simulink model "sf_newtons_cradle_vr"  (R2017b)
settings: Solver=ode45  StartTime=0.0  StopTime=inf  RelTol=1e-3
libraries: vrlib x3
settings Model: Creator=The MathWorks, Inc.  LastModifiedBy=The MathWorks, Inc.
settings DataIOCC: LimitDataPoints=on  SaveFormat=Array
settings OptimizationCC: BlockReduction=off  ExpressionDepthLimit=2147483647  InitFltsAndDblsToZero=on  LifeSpan=inf
settings DebuggingCC: UnderspecifiedInitializationDetection=Classic  MergeDetectMultiDrivingBlocksExec=none  SignalResolutionControl=TryResolveAllWithWarning  FcnCallInpInsideContextMsg=warning  StateNameClashWarn=warning  StrictBusMsg=Warning  SFUnexpectedBacktrackingDiag=warning  SFNoUnconditionalDefaultTransitionDiag=warning  SFExecutionAtInitializationDiag=none
settings HardwareCC: ProdBitPerPointer=32  ProdBitPerSizeT=32  ProdBitPerPtrDiffT=32  ProdLargestAtomicFloat=None  ProdIntDivRoundTo=Undefined  ProdEndianess=Unspecified  ProdWordSize=32  ProdHWDeviceType=32-bit Generic  TargetUnknown=on
settings ModelReferenceCC: PropagateSignalLabelsOutOfModel=off
settings SFSimCC: SFSimEcho=off  SimParseCustomCode=off
settings CodeAppCC: StateflowObjectComments=on
settings GRTTargetCC: TargetFcnLib=ansi_tfl_tmw_new.mat  TargetLangStandard=C89/C90 (ANSI)  GeneratePreprocessorConditionals=Disable all  CombineOutputUpdateFcns=off  GRTInterface=on
settings ConfigComp: CovMetricSettings=dw  CovHtmlReporting=on  CovSaveCumulativeToWorkspaceVar=on  CovSaveSingleToWorkspaceVar=on  CovExternalEMLEnable=off  CovSFcnEnable=off

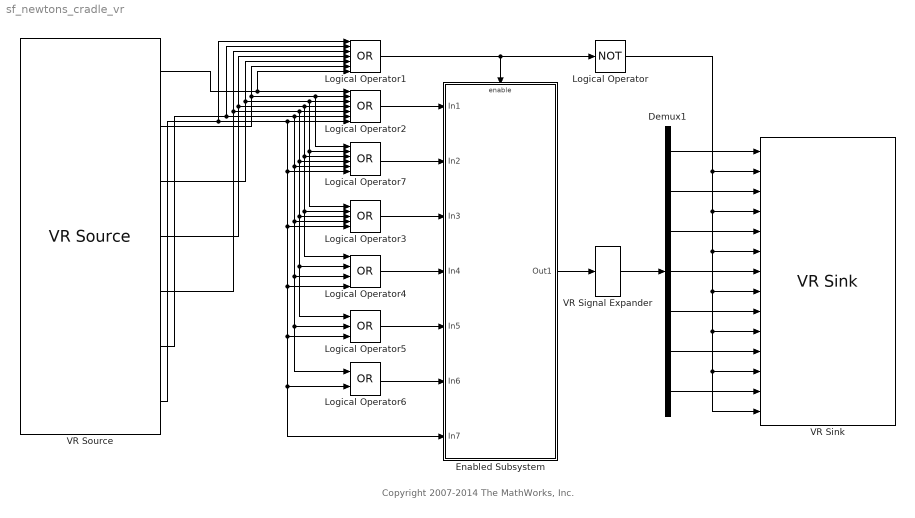
== system sf_newtons_cradle_vr ==
  note: Copyright 2007-2014 The MathWorks, Inc.
  Demux1 : Demux  Outputs=7
  Enabled Subsystem : Subsystem  TreatAsAtomicUnit=on
  Logical Operator : Logic  Operator=NOT  AllPortsSameDT=off  OutDataTypeStr=boolean
  Logical Operator1 : Logic  Operator=OR  Inputs=7  AllPortsSameDT=off  OutDataTypeStr=boolean
  Logical Operator2 : Logic  Operator=OR  Inputs=7  AllPortsSameDT=off  OutDataTypeStr=boolean
  Logical Operator3 : Logic  Operator=OR  Inputs=5  AllPortsSameDT=off  OutDataTypeStr=boolean
  Logical Operator4 : Logic  Operator=OR  Inputs=4  AllPortsSameDT=off  OutDataTypeStr=boolean
  Logical Operator5 : Logic  Operator=OR  Inputs=3  AllPortsSameDT=off  OutDataTypeStr=boolean
  Logical Operator6 : Logic  Operator=OR  AllPortsSameDT=off  OutDataTypeStr=boolean
  Logical Operator7 : Logic  Operator=OR  Inputs=6  AllPortsSameDT=off  OutDataTypeStr=boolean
  VR Signal Expander : vrlib/VR Signal Expander  outwidth=28  outidx=[4 8 12 16 20 24 28]
      settings: SourceProductName=Simulink 3D Animation  SourceProductBaseCode=VR
  VR Sink : vrlib/VR Sink  InstantiateOnLoad=on  SampleTime=0.01  ViewEnable=on  RemoteChange=off  RemoteView=off  FieldsWritten=Assembly1.ProtoRotation.4.1.1.double#Assembly1.ProtoEnabled.1.1.1.logical#Assembly2.ProtoRotation.4.1.1.double#Assembly2.ProtoEnabled.1.1.1.logical#Assembly3.ProtoRotation.4.1.1.double#Assembly3.ProtoEnabled.1.1.1.logical#Assembly4.ProtoRotation.4.1.1.double#Assembly4.ProtoEnabled.1.1.1.logical#Assembly5.ProtoRotation.4.1.1.double#Assembly5.ProtoEnabled.1.1.1.logical#Assembly6.ProtoRotation.4.1.1.double#Assembly6.ProtoEnabled.1.1.1.logical#Assembly7.ProtoRotation.4.1.1.double#Assembly7.ProtoEnabled.1.1.1.logical  WorldFileName=cradle.wrl  AutoView=off  VideoDimensions=[]  AllowVariableSize=off
      settings: SourceProductBaseCode=VR
  VR Source : vrlib/VR Source  InstantiateOnLoad=on  SampleTime=0.1  ViewEnable=on  RemoteChange=off  RemoteView=off  FieldsRead=Assembly1.ProtoIsActive.1.1.1.logical#Assembly2.ProtoIsActive.1.1.1.logical#Assembly3.ProtoIsActive.1.1.1.logical#Assembly4.ProtoIsActive.1.1.1.logical#Assembly5.ProtoIsActive.1.1.1.logical#Assembly6.ProtoIsActive.1.1.1.logical#Assembly7.ProtoIsActive.1.1.1.logical  WorldFileName=cradle.wrl  AutoView=off  VideoDimensions=[]  AllowVariableSize=off
      settings: SourceProductName=Simulink 3D Animation  SourceProductBaseCode=VR
  wires:
  Demux1/1 -> VR Sink/1
  Demux1/2 -> VR Sink/3
  Demux1/3 -> VR Sink/5
  Demux1/4 -> VR Sink/7
  Demux1/5 -> VR Sink/9
  Demux1/6 -> VR Sink/11
  Demux1/7 -> VR Sink/13
  Logical Operator/1 -> VR Sink/2, VR Sink/8, VR Sink/14, VR Sink/12, VR Sink/10, VR Sink/6, VR Sink/4
  VR Signal Expander/1 -> Demux1/1
  Logical Operator1/1 -> Logical Operator/1, Enabled Subsystem/Enable
  VR Source/1 -> Logical Operator1/7, Logical Operator2/1
  VR Source/2 -> Logical Operator1/6, Logical Operator2/2, Logical Operator7/1
  VR Source/3 -> Logical Operator1/5, Logical Operator3/1, Logical Operator7/2, Logical Operator2/3
  VR Source/4 -> Logical Operator1/4, Logical Operator4/1, Logical Operator3/2, Logical Operator7/3, Logical Operator2/4
  VR Source/5 -> Logical Operator1/3, Logical Operator5/1, Logical Operator4/2, Logical Operator3/3, Logical Operator7/4, Logical Operator2/5
  Logical Operator2/1 -> Enabled Subsystem/1(In1)
  Logical Operator7/1 -> Enabled Subsystem/2(In2)
  Logical Operator3/1 -> Enabled Subsystem/3(In3)
  Logical Operator4/1 -> Enabled Subsystem/4(In4)
  Logical Operator5/1 -> Enabled Subsystem/5(In5)
  Logical Operator6/1 -> Enabled Subsystem/6(In6)
  VR Source/6 -> Logical Operator1/2, Logical Operator6/1, Logical Operator5/2, Logical Operator4/3, Logical Operator3/4, Logical Operator7/5, Logical Operator2/6
  VR Source/7 -> Logical Operator1/1, Enabled Subsystem/7(In7), Logical Operator6/2, Logical Operator5/3, Logical Operator4/4, Logical Operator3/5, Logical Operator7/6, Logical Operator2/7
  Enabled Subsystem/1(Out1) -> VR Signal Expander/1

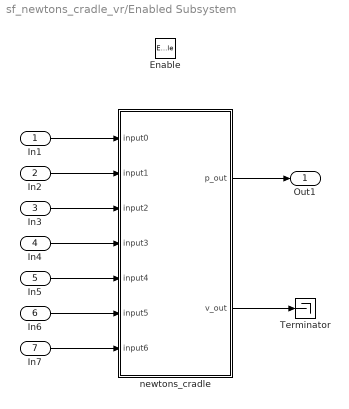
== system sf_newtons_cradle_vr/Enabled Subsystem ==
  In1 : Inport
  In2 : Inport  Port=2
  In3 : Inport  Port=3
  In4 : Inport  Port=4
  In5 : Inport  Port=5
  In6 : Inport  Port=6
  In7 : Inport  Port=7
  Enable : EnablePort
  Terminator : Terminator
  newtons_cradle : Stateflow chart  TreatAsAtomicUnit=on
  Out1 : Outport
  wires:
  newtons_cradle/2(v_out) -> Terminator/1
  newtons_cradle/1(p_out) -> Out1/1
  In3/1 -> newtons_cradle/3(input2)
  In4/1 -> newtons_cradle/4(input3)
  In2/1 -> newtons_cradle/2(input1)
  In1/1 -> newtons_cradle/1(input0)
  In5/1 -> newtons_cradle/5(input4)
  In6/1 -> newtons_cradle/6(input5)
  In7/1 -> newtons_cradle/7(input6)

== stateflow chart sf_newtons_cradle_vr/Enabled Subsystem/newtons_cradle ==
  settings: updateMethod=CONTINUOUS  initializeOutput=1
  state FreeDynamics
    du:
    p_out = p;
    v_out = v;
    p_dot = v;
    v_dot = -g/l*sin(p);
  state resetPositionsAndVelocities [function]
    (default) -> (junction 22) : {i=0;}
    (junction 22) -> (junction 24) [order 1] : [i < k-1]
    (junction 17) -> (junction 22) : {i++;}
    (junction 24) -> (junction 17) [order 2]
    (junction 24) -> (junction 17) [order 1] : [p[i] < p[i+1]]
        | {
        | // swap positions
        | tmp = p[i];
        | p[i] = p[i+1];
        | p[i+1] = tmp;
        | // swap velocities
        | tmp = v[i];
        | v[i] = v[i+1];
        | v[i+1] = tmp;
        | }
    (junction 22) -> (junction 23) [order 2]
  state collision = isCollisionPossible [function]
    (default) -> (junction 18) : {i=0;}
    (junction 18) -> (junction 20) [order 1] : [i < k-1]
    (junction 20) -> (junction 18) [order 2] : {i++;}
    (junction 18) -> (junction 19) [order 2] : {
        | collision = 0;
        | }
    (junction 20) -> (junction 21) [order 1] : [p[i] < p[i+1]]
        | {
        | collision = 1;
        | }
  (default) -> FreeDynamics : {
      | p = 0;
      | v = 0;
      |
      | p[0] = pi/3*input0;
      | p[1] = pi/3*input1;
      | p[2] = pi/3*input2;
      | p[3] = pi/3*input3;
      | p[4] = pi/3*input4;
      | p[5] = pi/3*input5;
      | p[6] = pi/3*input6;
      |
      | // uncomment the lines below to see
      | // some interesting behavior
      | // p[k-3] = -pi/6;
      | //p[k-2] = -pi/6;
      | // p[k-1] = -pi/6;
      | // v[0] = 2;
      | }
  FreeDynamics -> FreeDynamics : [isCollisionPossible()]
      | {resetPositionsAndVelocities();}
  data: i temporary double; tmp temporary double; collision function_output double; i temporary double; input0 input; p_out output double size=k; v_out output double size=k; g constant double =9.81; l constant double =1; pi constant double =3.141; p local double size=k; v local double size=k; k constant int32 =7; input1 input; input2 input; input3 input; input4 input; input5 input; input6 input
  data p settings: updateMethod=SF_CONTINUOUS_TIME_DATA
  data v settings: updateMethod=SF_CONTINUOUS_TIME_DATA
